simulink model "busBasics"  (R2022b)
settings: Solver=FixedStepAuto  StartTime=0.0  StopTime=10.0  FixedStep=0.01  RelTol=1e-3
InitFcn:
  | Ts = 0.01;
settings Model: Creator=System-10  LastModifiedBy=System-10

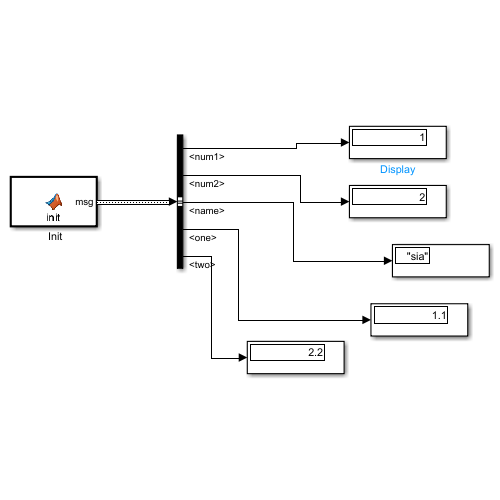
[thumbnail: Simulink's stored preview of the top-level diagram]
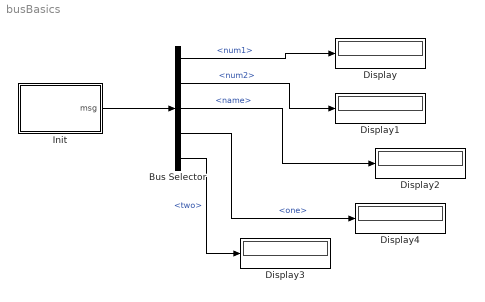
== system busBasics ==
  " Init" : MATLAB Function  TreatAsAtomicUnit=on
  Bus Selector : BusSelector  OutputSignals=num1,num2,name,Q.one,Q.two
  Display{,1..4} (5 alike) : Display
  wires:
  " Init"/1(msg) -> Bus Selector/1
  Bus Selector/1 -> Display/1  "<num1>"
  Bus Selector/2 -> Display1/1  "<num2>"
  Bus Selector/3 -> Display2/1  "<name>"
  Bus Selector/4 -> Display4/1  "<one>"
  Bus Selector/5 -> Display3/1  "<two>"

== matlab function busBasics/ Init ==
  settings: updateMethod=DISCRETE  sampleTime=Ts
  data: msg output Bus: TestBus
function msg = init
    msg.num1 = 1;
    msg.num2 = 2;
    msg.name = "sia";

    msg.Q.one = 1.1;
    msg.Q.two = 2.2;
end
